simulink model "model"  (R2023b)
settings: Solver=VariableStepAuto  StartTime=0.0  StopTime=10  RelTol=1e-3
values from neighbouring files (symbols this model uses):
  dt = 0.2    [config.m]
  l = size(C,1)    [config.m]    (also in mpc_coeffs.m)
  m = size(B,2)    [config.m]    (also in mpc_coeffs.m)
  n = size(A,2)    [config.m]    (also in mpc_coeffs.m)
  N = ceil(tf/dt)    [config.m]    (also in mpc_coeffs.m = params.N)
  sysc = ss(A,B,C,D)    [config.m]
  x0 = [1;0]    [config.m]
undefined symbols (not defined in the file or in its folder): MPC, MPC_compensated
settings Model: Creator=MPC5  LastModifiedBy=MPC5

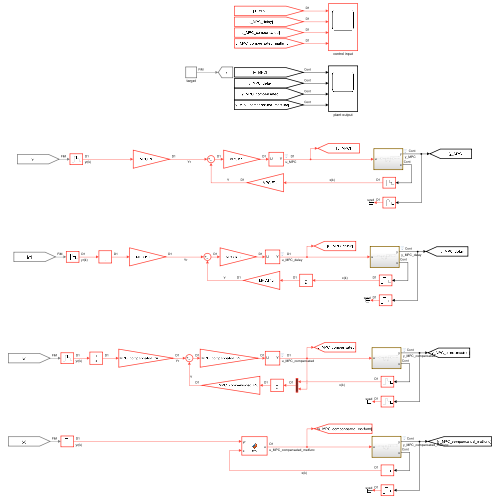
[thumbnail: Simulink's stored preview of the top-level diagram]
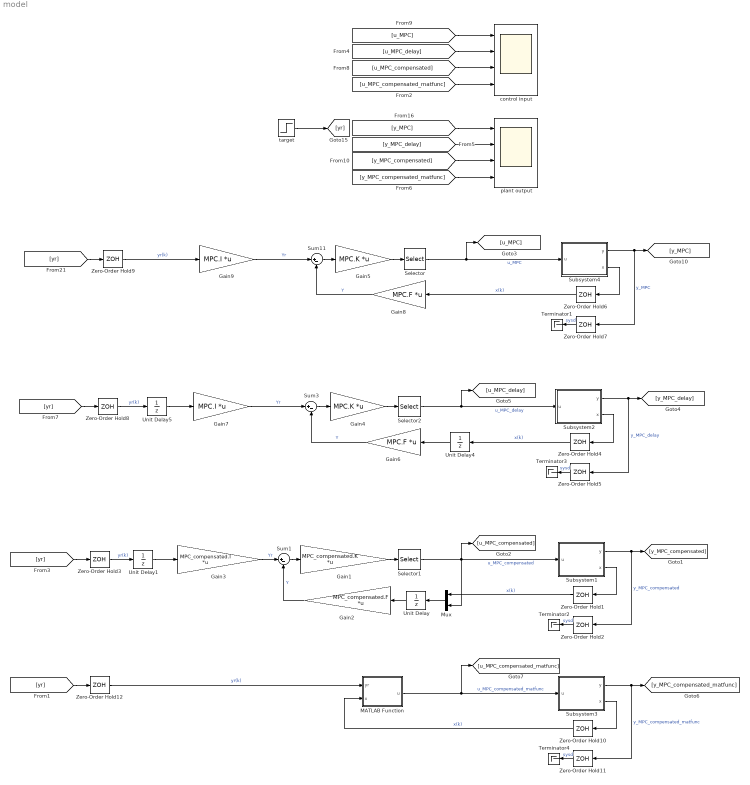
== system model ==
  Gain1 : Gain  Gain=MPC_compensated.K  Multiplication=Matrix(K*u)
  Gain2 : Gain  Gain=MPC_compensated.F  Multiplication=Matrix(K*u)
  Gain3 : Gain  Gain=MPC_compensated.I  Multiplication=Matrix(K*u)
  Gain4 : Gain  Gain=MPC.K  Multiplication=Matrix(K*u)
  Gain5 : Gain  Gain=MPC.K  Multiplication=Matrix(K*u)
  Gain6 : Gain  Gain=MPC.F  Multiplication=Matrix(K*u)
  Gain7 : Gain  Gain=MPC.I  Multiplication=Matrix(K*u)
  Gain8 : Gain  Gain=MPC.F  Multiplication=Matrix(K*u)
  Gain9 : Gain  Gain=MPC.I  Multiplication=Matrix(K*u)
  MATLAB Function : MATLAB Function  TreatAsAtomicUnit=on
  Mux : Mux  Inputs=2
  Selector : Selector  InputPortWidth=N  IndexOptions=Index vector (dialog)  Indices=1:m  OutputSizes=1
  Selector1 : Selector  InputPortWidth=m*(N-1)  IndexOptions=Index vector (dialog)  Indices=1:m  OutputSizes=1
  Selector2 : Selector  InputPortWidth=N  IndexOptions=Index vector (dialog)  Indices=1:m  OutputSizes=1
  Subsystem1 : Subsystem
  Subsystem2 : Subsystem
  Subsystem3 : Subsystem
  Subsystem4 : Subsystem
  Sum1 : Sum  Inputs=|+-
  Sum11 : Sum  Inputs=|+-
  Sum3 : Sum  Inputs=|+-
  Terminator{1..4} (4 alike) : Terminator
  Unit Delay{,1,4..5} (4 alike) : UnitDelay  SampleTime=-1  HasFrameUpgradeWarning=on
  Zero-Order Hold{1..12} (12 alike) : ZeroOrderHold  SampleTime=dt
  control input : Scope  NumInputPorts=4
  plant output : Scope  NumInputPorts=4
  target : Step  Time=5  SampleTime=0
  wires:
  Subsystem4/2(x) -> Zero-Order Hold6/1
  Subsystem4/1(y) -> [y_MPC], Zero-Order Hold7/1  "y_MPC"
  Sum11/1 -> Gain5/1
  Zero-Order Hold6/1 -> Gain8/1  "x(k)"
  Selector/1 -> Subsystem4/1(u), [u_MPC]  "u_MPC"
  Zero-Order Hold7/1 -> Terminator1/1  "sysd"
  [u_MPC] -> control input/1
  [u_MPC_delay] -> control input/2
  [u_MPC_compensated] -> control input/3
  [y_MPC] -> plant output/1
  [y_MPC_delay] -> plant output/2
  [y_MPC_compensated] -> plant output/3
  Gain8/1 -> Sum11/2  "Y"
  Gain9/1 -> Sum11/1  "Yr"
  [yr] -> Zero-Order Hold9/1
  target/1 -> [yr]
  Gain5/1 -> Selector/1
  Zero-Order Hold9/1 -> Gain9/1  "yr(k)"
  Zero-Order Hold2/1 -> Terminator2/1  "sysd"
  Selector1/1 -> Subsystem1/1(u), Mux/2, [u_MPC_compensated]  "u_MPC_compensated"
  Zero-Order Hold1/1 -> Mux/1  "x(k)"
  Subsystem1/2(x) -> Zero-Order Hold1/1
  Sum1/1 -> Gain1/1
  Gain3/1 -> Sum1/1  "Yr"
  [yr] -> Zero-Order Hold3/1
  Zero-Order Hold3/1 -> Unit Delay1/1  "yr(k)"
  Gain1/1 -> Selector1/1
  Subsystem1/1(y) -> [y_MPC_compensated], Zero-Order Hold2/1  "y_MPC_compensated"
  Gain2/1 -> Sum1/2  "Y"
  Mux/1 -> Unit Delay/1
  Unit Delay/1 -> Gain2/1
  Unit Delay1/1 -> Gain3/1
  Unit Delay5/1 -> Gain7/1
  Unit Delay4/1 -> Gain6/1
  Zero-Order Hold8/1 -> Unit Delay5/1  "yr(k)"
  Gain4/1 -> Selector2/1
  [yr] -> Zero-Order Hold8/1
  Gain7/1 -> Sum3/1  "Yr"
  Gain6/1 -> Sum3/2  "Y"
  Zero-Order Hold5/1 -> Terminator3/1  "sysd"
  Selector2/1 -> Subsystem2/1(u), [u_MPC_delay]  "u_MPC_delay"
  Zero-Order Hold4/1 -> Unit Delay4/1  "x(k)"
  Sum3/1 -> Gain4/1
  Subsystem2/1(y) -> Zero-Order Hold5/1, [y_MPC_delay]  "y_MPC_delay"
  Subsystem2/2(x) -> Zero-Order Hold4/1
  Subsystem3/1(y) -> Zero-Order Hold11/1, [y_MPC_compensated_matfunc]  "y_MPC_compensated_matfunc"
  Zero-Order Hold12/1 -> MATLAB Function/1(yr)  "yr(k)"
  [yr] -> Zero-Order Hold12/1
  Subsystem3/2(x) -> Zero-Order Hold10/1
  Zero-Order Hold10/1 -> MATLAB Function/2(x)  "x(k)"
  MATLAB Function/1(u) -> [u_MPC_compensated_matfunc], Subsystem3/1(u)  "u_MPC_compensated_matfunc"
  Zero-Order Hold11/1 -> Terminator4/1  "sysd"
  [u_MPC_compensated_matfunc] -> control input/4
  [y_MPC_compensated_matfunc] -> plant output/4

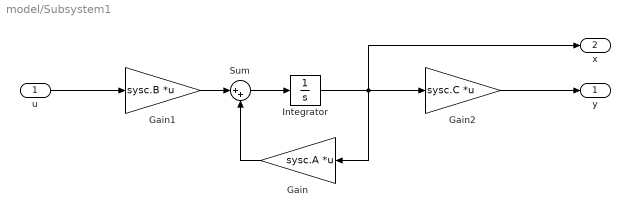
== system model/Subsystem1 ==
  u : Inport
  Gain : Gain  Gain=sysc.A  Multiplication=Matrix(K*u)
  Gain1 : Gain  Gain=sysc.B  Multiplication=Matrix(K*u)
  Gain2 : Gain  Gain=sysc.C  Multiplication=Matrix(K*u)
  Integrator : Integrator  InitialCondition=x0
  Sum : Sum  Inputs=|++
  y : Outport
  x : Outport  Port=2
  wires:
  Gain2/1 -> y/1
  Gain1/1 -> Sum/1
  Sum/1 -> Integrator/1
  Integrator/1 -> Gain/1, Gain2/1, x/1
  Gain/1 -> Sum/2
  u/1 -> Gain1/1

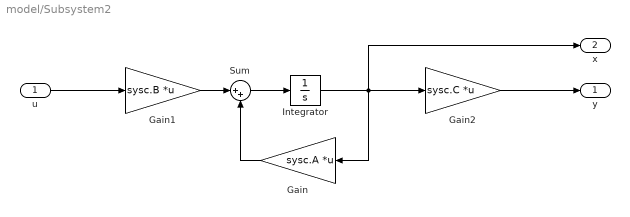
== system model/Subsystem2 ==
  u : Inport
  Gain : Gain  Gain=sysc.A  Multiplication=Matrix(K*u)
  Gain1 : Gain  Gain=sysc.B  Multiplication=Matrix(K*u)
  Gain2 : Gain  Gain=sysc.C  Multiplication=Matrix(K*u)
  Integrator : Integrator  InitialCondition=x0
  Sum : Sum  Inputs=|++
  y : Outport
  x : Outport  Port=2
  wires:
  u/1 -> Gain1/1
  Gain/1 -> Sum/2
  Integrator/1 -> x/1, Gain2/1, Gain/1
  Sum/1 -> Integrator/1
  Gain1/1 -> Sum/1
  Gain2/1 -> y/1

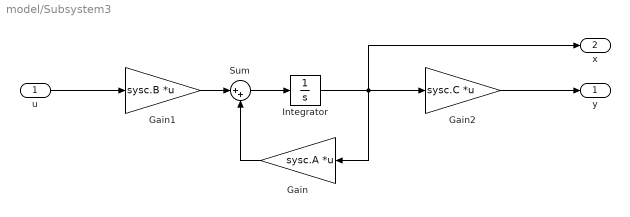
== system model/Subsystem3 ==
  u : Inport
  Gain : Gain  Gain=sysc.A  Multiplication=Matrix(K*u)
  Gain1 : Gain  Gain=sysc.B  Multiplication=Matrix(K*u)
  Gain2 : Gain  Gain=sysc.C  Multiplication=Matrix(K*u)
  Integrator : Integrator  InitialCondition=x0
  Sum : Sum  Inputs=|++
  y : Outport
  x : Outport  Port=2
  wires:
  u/1 -> Gain1/1
  Gain/1 -> Sum/2
  Integrator/1 -> x/1, Gain2/1, Gain/1
  Sum/1 -> Integrator/1
  Gain1/1 -> Sum/1
  Gain2/1 -> y/1

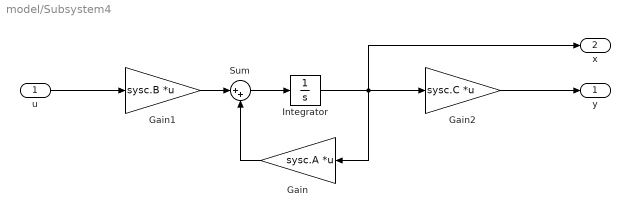
== system model/Subsystem4 ==
  u : Inport
  Gain : Gain  Gain=sysc.A  Multiplication=Matrix(K*u)
  Gain1 : Gain  Gain=sysc.B  Multiplication=Matrix(K*u)
  Gain2 : Gain  Gain=sysc.C  Multiplication=Matrix(K*u)
  Integrator : Integrator  InitialCondition=x0
  Sum : Sum  Inputs=|++
  y : Outport
  x : Outport  Port=2
  wires:
  Gain2/1 -> y/1
  Gain1/1 -> Sum/1
  Sum/1 -> Integrator/1
  Integrator/1 -> Gain/1, Gain2/1, x/1
  Gain/1 -> Sum/2
  u/1 -> Gain1/1

== matlab function model/MATLAB Function ==
  data: yr input size=l; u output size=m; x input size=n; MPC_compensated parameter; n parameter; m parameter; l parameter
function u = fcn(yr,x,MPC_compensated, n, m, l)
    persistent u_;
    if (isempty(u_))
        u_ = zeros(m,1);
    end

    u = u_;

    Yr = MPC_compensated.I*yr;
    Y = MPC_compensated.F*[x;u];
    tmp = MPC_compensated.K*(Yr - Y);
    u_ = tmp(1:m);
end
